simulink model "Projet_Final"  (R2024a)
settings: Solver=FixedStepAuto  StartTime=0.0  StopTime=6  FixedStep=Ts  RelTol=1e-3
values from neighbouring files (symbols this model uses):
  A1 = 0.548    [Parameters.m]
  A2 = 116    [Parameters.m]
  A3 = 0.4    [Parameters.m]
  A4 = 5    [Parameters.m]
  A5 = -21    [Parameters.m]
  A6 = 0.0068    [Parameters.m]
  C_Bat = 1e-3    (= 0.001)    [Parameters.m]    (also in Params_Battery_converter.m)
  C_dc = 4.5e-3    (= 0.0045)    [Parameters.m]
  f = 50    [Parameters.m]
  F = 0.0004924    [Parameters.m]
  G = 6.24    [Parameters.m]
  J = J_PMSG    (= 0.2227)    [Parameters.m]
  J_PMSG = 0.2227    [Parameters.m]
  ki_Ibat = 550    [Parameters.m]    (also in Params_Battery_converter.m)
  ki_id_grid = 225    [Parameters.m]
  ki_iq_grid = ki_id_grid    (= 225)    [Parameters.m]
  ki_isd = 13800    [Parameters.m]
  ki_omega = 0.6873    [Parameters.m]
  ki_PLL = 3200    [Parameters.m]
  ki_Q = 0.05    [Parameters.m]
  ki_vdc = C_dc * W_vdc^2    (= 28.8)    [Parameters.m]
  kp_Ibat = 6.28    [Parameters.m]    (also in Params_Battery_converter.m)
  kp_id_grid = 4.5    [Parameters.m]
  kp_iq_grid = kp_id_grid    (= 4.5)    [Parameters.m]
  kp_isd = 2.75    [Parameters.m]
  kp_omega = 3.108    [Parameters.m]
  kp_PLL = 180    [Parameters.m]
  kp_Q = 0.0005    [Parameters.m]
  kp_vdc = 2 * C_dc * W_vdc    (= 0.72)    [Parameters.m]
  Kt = 1.5 * p * Phi_r    (= 0.7164)    [Parameters.m]
  L_Bat = 2e-3    (= 0.002)    [Parameters.m]    (also in Params_Battery_converter.m)
  Lf = 8e-3    (= 0.008)    [Parameters.m]
  Ls = 0.000395    [Parameters.m]
  p = 4    [Parameters.m]
  Phi_r = 0.1194    [Parameters.m]
  R = 3.96    [Parameters.m]
  Rf = 0.01    [Parameters.m]
  rho = 1.225    [Parameters.m]
  Rs = 0.0485    [Parameters.m]
  S = pi*R^2    (= 49.2651993565)    [Parameters.m]
  Ts = 1e-6    (= 1e-06)    [Parameters.m]
  Vdc_ref = 700    [Parameters.m]    (also in Params_Battery_converter.m)
undefined symbols (not defined in the file or in its folder): Ion, Lithium
libraries: spsSeriesRLCBranchLib x19, slpidlib x11, spsMeanLib x6, spsThreePhaseVIMeasurementLib x6, spsThreePhaseBreakerLib x6, spsIdealSwitchLib x4, spsThreePhaseParallelRLCLoadLib x4, spsCurrentMeasurementLib x3, eeTransforms x3, spsPWMGenerator2LevelLib x3, spsVoltageMeasurementLib x3, spsUniversalBridgeLib x2
(part 1 of 3)
settings Model: SimulationMode=accelerator  Creator=K Edd Edd  LastModifiedBy=K Edd Edd
settings DataIOCC: SignalLogging=off  DSMLogging=off  ReturnWorkspaceOutputs=off

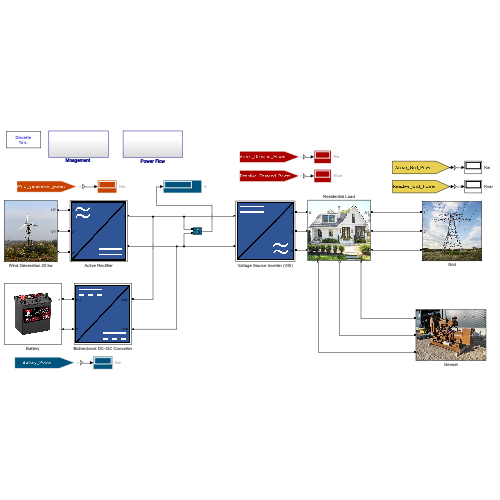
[thumbnail: Simulink's stored preview of the top-level diagram]
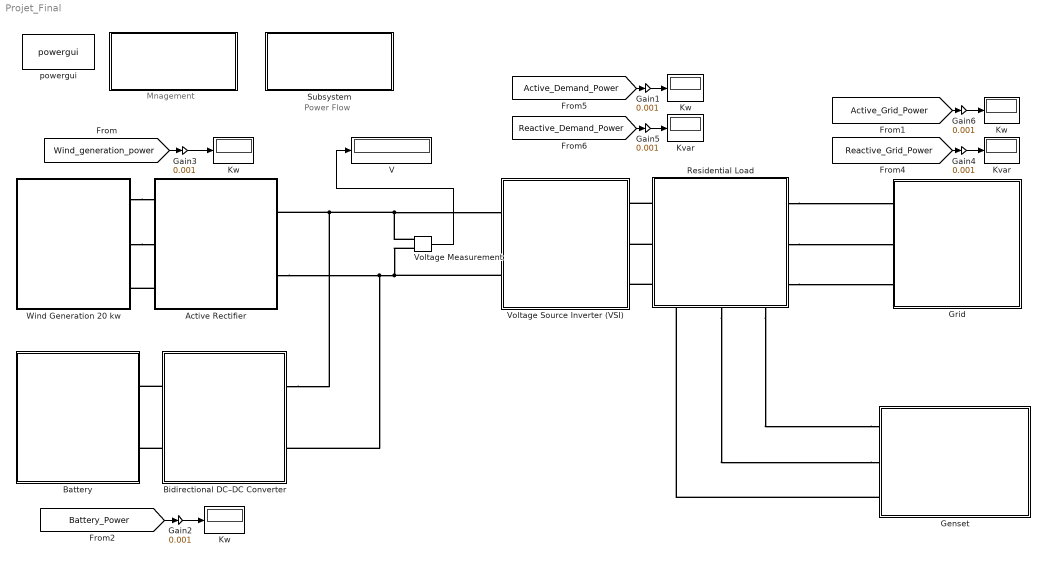
== system Projet_Final ==
  note: Mnagement
  note: Power Flow
  "    " : Subsystem
  Active Rectifier : Subsystem
      mask Display: image('AC-DC converter.png');
  Battery : Subsystem
      mask Display: image('Batterie.jpg', [0,0,0,0,90,90]);
  Bidirectional DC–DC Converter : Subsystem
      mask Display: image('DC-DC converter.png');
  Gain{1..6} (6 alike) : Gain  Gain=0.001
  Genset : Subsystem
      mask Display: image('Cummins-140-kVA-Leroy-Somer-generatorset-Netherlands_8218_1779787131390.jpg');
  Grid : Subsystem
      mask Display: image('df15ac89cc852b7c79e11306f20382d1.jpg');
  Kvar : Display
      settings: Format=bank
  "Kvar  " : Display
      settings: Format=bank
  Kw : Display
      settings: Format=bank
  "Kw  " : Display
      settings: Format=bank
  "Kw   " : Display
      settings: Format=bank
  "Kw    " : Display
      settings: Format=bank
  Residential Load : Subsystem
      settings: PortSchema="{\"entries\":[{\"content\":{\"sides\":[{\"content\":{\"connectorIds\":[\"LConn1\",\"LConn2\",\"LConn3\"]},\"type\":\"ConnectorPlacement.EquallySpacedRectSide\",\"uuid\":\"15385e33-3697-4ec0-8f2e-b1014489e4b6\"},{\"content\":{\"connectorIds\":[\"RConn1\",\"RConn2\",\"RConn3\"],\"side\":\"RIGHT\"},\"type\":\"ConnectorPlacement.EquallySpacedRectSide\",\"uuid\":\"d6a0931e-fc44-44c1-903e-3bbebba5ba41\"},{\"content\":{\"side\":\"TOP\"},\"type\":\"ConnectorPlacement.EquallySpacedRectSide\",\"uuid\":\"1d080c2c-00e5-4060-a5ce-b97d059839f9\"},{\"content\":{\"connectorIds\":[\"RConn4\",\"RConn5\",\"RConn6\"],\"side\":\"BOTTOM\"},\"type\":\"ConnectorPlacement.EquallySpacedRectSide\",\"uuid\":\"92a56d4a-46c7-4b37-87a4-59d3c02e3066\"}]},\"type\":\"ConnectorPlacement.EquallySpacedConnector\",\"uuid\":\"422ce4c9-7dd0-497d-8c7c-a95a054bb062\"}],\"packageUris\":[\"http://schema.mathworks.com/mf0/Connector/R2020b\"],\"version\":\"1.0\"}"
      mask Display: image('home.jpeg');
  Subsystem : Subsystem
  V : Display
      settings: Format=bank
  Voltage Measurement : spsVoltageMeasurementLib/Voltage Measurement  PhasorSimulation=off  OutputType=Complex  PSBequivalent=0
  Voltage Source Inverter (VSI) : Subsystem
      mask Display: image('DC-AC converter.png');
  Wind Generation 20 kw : Subsystem
      mask Display: image('Wind_Turbine.jpg');
  powergui : spspowerguiLib/powergui  Priority=1  SimulationMode=Discrete  SampleTime=Ts  frequency=60  Iterations=50  frequencyindice=0  Pbase=100e6  ErrMax=1e-4  UnitsV=kV  UnitsW=MW  buscounter=0  FunctionMessages=off  echomessages=off  EnableUseOfTLC=off  CurrentSourceSwitches=off  DisableSnubberDevices=off  DisableRonSwitches=off  DisableVfSwitches=off  DisplayEquations=off  AutomaticDiscreteSolvers=off  SolverType=Tustin/Backward Euler (TBE)  Interpol=off  ExternalGateDelay=off  methode=off  Ts=100  x0status=blocks  SPID=on  SwTol=0  HookPort=off  NonlinearTolerance=1e-4  nMaxIteration=100  ContinueOnMaxIteration=off  RestoreLinks=warning  ResistiveCurrentMeasurement=off  Frange=[0:2:500]  Ylog=off  Xlog=on  ShowGrid=off  save=off  variable=ZData  structure=0  ZoomFFT=off  StartTime=0.0  cycles=1  DisplayStyle=1  fundamental=60  FreqAxis=off  MaxFrequency=1000  frequencyindicesteady=1  RmsSteady=1  display=off
  wires:
  Voltage Measurement/1 -> V/1
  Gain3/1 -> Kw/1
  [Wind_generation_power] -> Gain3/1
  Gain2/1 -> "Kw  "/1
  [Battery_Power] -> Gain2/1
  [Reactive_Grid_Power] -> Gain4/1
  [Active_Grid_Power] -> Gain6/1
  Gain5/1 -> Kvar/1
  Gain1/1 -> "Kw   "/1
  [Active_Demand_Power] -> Gain1/1
  [Reactive_Demand_Power] -> Gain5/1
  Gain6/1 -> "Kw    "/1
  Gain4/1 -> "Kvar  "/1
  connections:
  Wind Generation 20 kw/RConn1 -- Active Rectifier/LConn1
  Active Rectifier/LConn3 -- Wind Generation 20 kw/RConn3
  Residential Load/RConn3 -- Grid/LConn3
  Voltage Measurement/LConn1 -- Voltage Source Inverter (VSI)/LConn1 -- Bidirectional DC–DC Converter/LConn1 -- Active Rectifier/RConn1
  Voltage Source Inverter (VSI)/LConn2 -- Active Rectifier/RConn2 -- Bidirectional DC–DC Converter/LConn2 -- Voltage Measurement/LConn2
  Wind Generation 20 kw/RConn2 -- Active Rectifier/LConn2
  Bidirectional DC–DC Converter/RConn1 -- Battery/RConn1
  Bidirectional DC–DC Converter/RConn2 -- Battery/RConn2
  Residential Load/RConn1 -- Grid/LConn1
  Residential Load/RConn2 -- Grid/LConn2
  Residential Load/LConn2 -- Voltage Source Inverter (VSI)/RConn2
  Residential Load/LConn1 -- Voltage Source Inverter (VSI)/RConn1
  Residential Load/LConn3 -- Voltage Source Inverter (VSI)/RConn3
  Genset/RConn3 -- Residential Load/RConn4
  Residential Load/RConn5 -- Genset/RConn2
  Residential Load/RConn6 -- Genset/RConn1

== system Projet_Final/     ==
  Constant{,1..3,5} (5 alike) : Constant
  Constant6 : Constant  Value=0
  tag scope: Cmd_Breaker_Disel=global, Cmd_Breaker_Grid=global, Enable_PWM_GSC=global, Enable_PWM_MSC=global, Enable_Sync=global, Mode_Injection_GSC=global
  wires:
  Constant/1 -> [Cmd_Breaker_Grid]
  Constant1/1 -> [Enable_PWM_GSC]
  Constant2/1 -> [Mode_Injection_GSC]
  Constant3/1 -> [Enable_PWM_MSC]
  Constant6/1 -> [Cmd_Breaker_Disel]
  Constant5/1 -> [Enable_Sync]

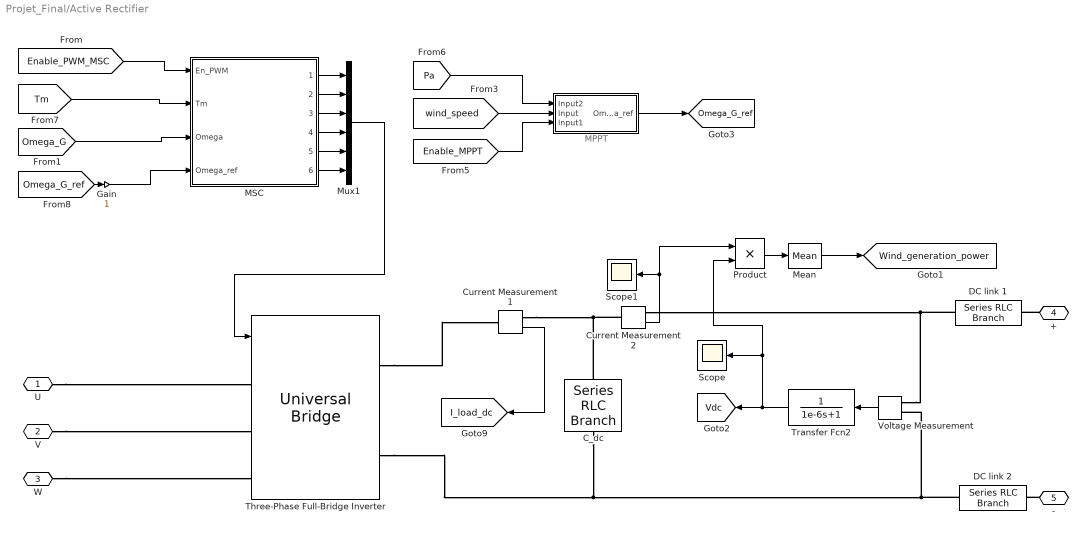
== system Projet_Final/Active Rectifier ==
  note: MPPT
  "      " : Subsystem
  C_dc : spsSeriesRLCBranchLib/Series RLC Branch  LConnTagsString=__new0  RConnTagsString=__new0  BranchType=C  Resistance=0  Inductance=1e-3  SetiL0=off  InitialCurrent=0  Capacitance=C_dc  Setx0=on  InitialVoltage=Vdc_ref  Measurements=None
  Current Measurement1 : spsCurrentMeasurementLib/Current Measurement  PhasorSimulation=off  OutputType=Complex  PSBequivalent=0
  Current Measurement2 : spsCurrentMeasurementLib/Current Measurement  PhasorSimulation=off  OutputType=Complex  PSBequivalent=0
  DC link 1 : spsSeriesRLCBranchLib/Series RLC Branch  LConnTagsString=__new0  RConnTagsString=__new0  BranchType=RL  Resistance=0.01  Inductance=1e-12  SetiL0=off  InitialCurrent=0  Capacitance=C_dc  Setx0=on  InitialVoltage=Vdc_ref  Measurements=None
  DC link 2 : spsSeriesRLCBranchLib/Series RLC Branch  LConnTagsString=__new0  RConnTagsString=__new0  BranchType=RL  Resistance=0.01  Inductance=1e-12  SetiL0=off  InitialCurrent=0  Capacitance=C_dc  Setx0=on  InitialVoltage=Vdc_ref  Measurements=None
  Gain : Gain
  MSC : Subsystem
      settings: PortSchema="{\"entries\":[{\"content\":{\"sides\":[{\"content\":{},\"type\":\"ConnectorPlacement.EquallySpacedRectSide\",\"uuid\":\"68bdff09-e8ec-4d6d-b05e-55201ee357f5\"},{\"content\":{\"side\":\"RIGHT\"},\"type\":\"ConnectorPlacement.EquallySpacedRectSide\",\"uuid\":\"a14a2bca-9db8-408e-b5bf-8e3869a2fb13\"},{\"content\":{\"connectorIds\":[\"Out1\",\"Out2\",\"Out3\",\"Out4\",\"Out5\",\"Out6\"],\"side\":\"TOP\"},\"type\":\"ConnectorPlacement.EquallySpacedRectSide\",\"uuid\":\"600d12f1-b4e8-4864-955c-a539efb19c99\"},{\"content\":{\"connectorIds\":[\"In1\",\"In2\",\"In3\",\"In4\"],\"side\":\"BOTTOM\"},\"type\":\"ConnectorPlacement.EquallySpacedRectSide\",\"uuid\":\"fe719057-0520-4d41-a82f-92eb49034055\"}]},\"type\":\"ConnectorPlacement.EquallySpacedConnector\",\"uuid\":\"05b2b3d9-6bdc-4d72-9457-a6c68afa543f\"}],\"packageUris\":[\"http://schema.mathworks.com/mf0/Connector/R2020b\"],\"version\":\"1.0\"}"
      mask Display: image('Cotroller.jpg', [0,0,0,0,70,70]);
  Mean : spsMeanLib/Mean  Freq=50  Vinit=0  Ts=0
  Mux1 : Mux  Inputs=6
  Product : Product
  Scope : Scope
  Scope1 : Scope
  Three-Phase Full-Bridge Inverter : spsUniversalBridgeLib/Universal Bridge  Arms=3  SnubberResistance=1e7  SnubberCapacitance=inf  Device=IGBT / Diodes  Ron=1e-2  Lon=0  ForwardVoltages="[  0  0  ]"  ForwardVoltage=0  GTOparameters=[ 10e-6 , 20e-6 ]  IGBTparameters=[ 0 , 0 ]  Measurements=None  Measurements_2=None  converterType=Rectifier
  Transfer Fcn2 : TransferFcn  Denominator=[1e-6 1]
  Voltage Measurement : spsVoltageMeasurementLib/Voltage Measurement  PhasorSimulation=off  OutputType=Complex  PSBequivalent=0
  U : PMIOPort  Side=Left
  V : PMIOPort  Port=2  Side=Left
  W : PMIOPort  Port=3  Side=Left
  + : PMIOPort  Port=4  Side=Right
  - : PMIOPort  Port=5  Side=Right
  tag scope: I_load_dc=global, Omega_G_ref=global, Vdc=global, Wind_generation_power=global
  wires:
  Mux1/1 -> Three-Phase Full-Bridge Inverter/1
  [Omega_G_ref] -> Gain/1
  [Tm] -> MSC/2(Tm)
  MSC/3("   ") -> Mux1/3
  MSC/1(" ") -> Mux1/1
  MSC/4("    ") -> Mux1/4
  MSC/6("       ") -> Mux1/6
  MSC/5("     ") -> Mux1/5
  [Omega_G] -> MSC/3(Omega)
  MSC/2("  ") -> Mux1/2
  Voltage Measurement/1 -> Transfer Fcn2/1
  Current Measurement2/1 -> Scope1/1, Product/1
  Current Measurement1/1 -> [I_load_dc]
  Product/1 -> Mean/1
  Mean/1 -> [Wind_generation_power]
  [Enable_PWM_MSC] -> MSC/1(En_PWM)
  "      "/1(Omega_ref) -> [Omega_G_ref]
  [wind_speed] -> "      "/2(Input)
  [Enable_MPPT] -> "      "/3(Input1)
  [Pa] -> "      "/1(Input2)
  Transfer Fcn2/1 -> [Vdc], Scope/1, Product/2
  Gain/1 -> MSC/4(Omega_ref)
  connections:
  V/RConn1 -- Three-Phase Full-Bridge Inverter/LConn2
  U/RConn1 -- Three-Phase Full-Bridge Inverter/LConn1
  W/RConn1 -- Three-Phase Full-Bridge Inverter/LConn3
  C_dc/RConn1 -- Three-Phase Full-Bridge Inverter/RConn2 -- DC link 2/LConn1 -- Voltage Measurement/LConn2
  Current Measurement2/LConn1 -- C_dc/LConn1 -- Current Measurement1/RConn1
  Three-Phase Full-Bridge Inverter/RConn1 -- Current Measurement1/LConn1
  Voltage Measurement/LConn1 -- DC link 1/LConn1 -- Current Measurement2/RConn1
  +/RConn1 -- DC link 1/RConn1
  -/RConn1 -- DC link 2/RConn1

== system Projet_Final/Battery ==
  Battery Status : Scope  NumInputPorts=4
  Battery1 : spsBatteryLib/Battery  BatType=Lithium-Ion  ShowTempParam=off  ThermalPreset=no  ShowAgeParam=off  NomV=450  NomQ=40  SOC=70  Batt_Tr=0.2  PresetModel=on  MaxQ=40  MinV=337.5  FullV=523.7942  Dis_rate=17.3913  R=0.1125  Normal_OP=36.1739  expZone="[486.1736      1.965217]"  current=[1.5 3]  Units=Ampere-hour  Tci=20  NomT=25  T2=0  MaxQ2=2.208  FullV2=3.45  Normal_OP2=2.8  expZone2="[3.22        0.23]"  Rca=0.6  ti=1000  Dp=0  Neq0=0  Tsim=1e6  Ta1=25  Qeol=5.4*0.9  Reol=0.013333*1.2  Char_age=[2.3478, 3]  Dis_age=[2.3478, 10]  N1=1500  N2=10500  N3=1000  N4=1400  Ta2=45  N5=950
      settings: LibrarySourceBlock=electricdrivelib/Extra Sources/Battery
  Bus Selector : BusSelector  OutputSignals=SOC (%),Current (A),Voltage (V)
  Display4 : Display
      settings: Format=bank
  Product1 : Product  RndMeth=Zero
  + : PMIOPort  Side=Right
  - : PMIOPort  Port=2  Side=Right
  tag scope: SOC=global
  wires:
  Product1/1 -> Battery Status/4  "Power_Battery[W]"
  Bus Selector/2 -> Product1/1, Battery Status/2  "<Current (A)>"
  Battery1/1 -> Bus Selector/1
  Bus Selector/3 -> Product1/2, Battery Status/3  "<Voltage (V)>"
  Bus Selector/1 -> Display4/1, [SOC], Battery Status/1  "<SOC (%)>"
  connections:
  Battery1/LConn2 -- -/RConn1
  Battery1/LConn1 -- +/RConn1

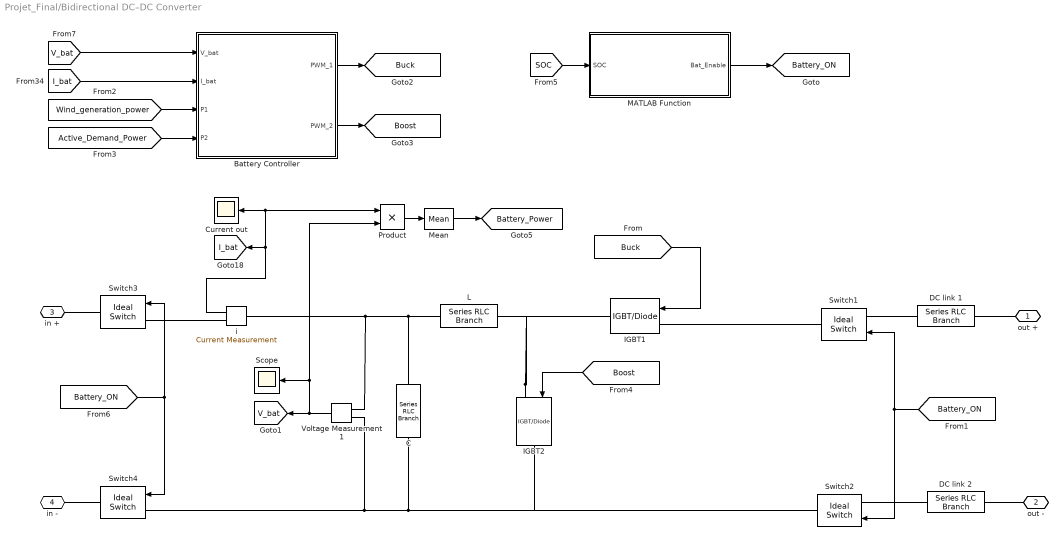
== system Projet_Final/Bidirectional DC–DC Converter ==
  Battery Controller : Subsystem
      mask Display: image('uC.png', [0,0,0,0,70,70]);
  C : spsSeriesRLCBranchLib/Series RLC Branch  LConnTagsString=__new0  RConnTagsString=__new0  BranchType=RC  Resistance=0.00001  Inductance=1e-3  SetiL0=off  InitialCurrent=0  Capacitance=C_Bat  Setx0=off  InitialVoltage=0  Measurements=None
  Current out : Scope
  DC link 1 : spsSeriesRLCBranchLib/Series RLC Branch  LConnTagsString=__new0  RConnTagsString=__new0  BranchType=RL  Resistance=0.01  Inductance=1e-12  SetiL0=off  InitialCurrent=0  Capacitance=C_dc  Setx0=on  InitialVoltage=Vdc_ref  Measurements=None
  DC link 2 : spsSeriesRLCBranchLib/Series RLC Branch  LConnTagsString=__new0  RConnTagsString=__new0  BranchType=RL  Resistance=0.01  Inductance=1e-12  SetiL0=off  InitialCurrent=0  Capacitance=C_dc  Setx0=on  InitialVoltage=Vdc_ref  Measurements=None
  IGBT1 : spsIGBTDiodeLib/IGBT//Diode  Ron=1e-3  Rs=1e5  Cs=inf  Measurements=off
  IGBT2 : spsIGBTDiodeLib/IGBT//Diode  Ron=1e-3  Rs=1e5  Cs=inf  Measurements=off
  L : spsSeriesRLCBranchLib/Series RLC Branch  LConnTagsString=__new0  RConnTagsString=__new0  BranchType=RL  Resistance=0.00001  Inductance=L_Bat  SetiL0=off  InitialCurrent=0  Capacitance=1000e-6  Setx0=off  InitialVoltage=0  Measurements=None
  MATLAB Function : MATLAB Function  TreatAsAtomicUnit=on
  Mean : spsMeanLib/Mean  Freq=50  Vinit=0  Ts=0
  Product : Product
  Scope : Scope
  Switch{1..4} (4 alike) : spsIdealSwitchLib/Ideal Switch  Ron=0.001  Lon=0  IC=0  Rs=1e6  Cs=inf  Measurements=off
  Voltage Measurement1 : spsVoltageMeasurementLib/Voltage Measurement  PhasorSimulation=off  OutputType=Complex  PSBequivalent=0
  i : spsCurrentMeasurementLib/Current Measurement  PhasorSimulation=off  OutputType=Complex  PSBequivalent=0
  out + : PMIOPort  Side=Left
  out - : PMIOPort  Port=2  Side=Left
  in + : PMIOPort  Port=3  Side=Right
  in - : PMIOPort  Port=4  Side=Right
  tag scope: Battery_ON=global, Battery_Power=global, Boost=global, Buck=global, I_bat=global, V_bat=global
  wires:
  [Buck] -> IGBT1/1
  MATLAB Function/1(Bat_Enable) -> [Battery_ON]
  [Wind_generation_power] -> Battery Controller/3(P1)
  Battery Controller/1(PWM_1) -> [Buck]
  [Battery_ON] -> Switch4/1, Switch3/1
  Mean/1 -> [Battery_Power]
  Battery Controller/2(PWM_2) -> [Boost]
  [Active_Demand_Power] -> Battery Controller/4(P2)
  Product/1 -> Mean/1
  [Boost] -> IGBT2/1
  [I_bat] -> Battery Controller/2(I_bat)
  Voltage Measurement1/1 -> Product/2, Scope/1, [V_bat]
  [Battery_ON] -> Switch1/1, Switch2/1
  [V_bat] -> Battery Controller/1(V_bat)
  [SOC] -> MATLAB Function/1(SOC)
  i/1 -> Product/1, Current out/1, [I_bat]
  connections:
  Switch3/RConn1 -- in +/RConn1
  Switch4/RConn1 -- in -/RConn1
  i/RConn1 -- Switch3/LConn1
  IGBT2/LConn1 -- L/RConn1 -- IGBT1/RConn1
  IGBT1/LConn1 -- Switch1/RConn1
  Voltage Measurement1/LConn1 -- C/LConn1 -- L/LConn1 -- i/LConn1
  DC link 1/RConn1 -- out +/RConn1
  DC link 2/LConn1 -- Switch2/LConn1
  Voltage Measurement1/LConn2 -- Switch2/RConn1 -- IGBT2/RConn1 -- C/RConn1 -- Switch4/LConn1
  Switch1/LConn1 -- DC link 1/LConn1
  out -/RConn1 -- DC link 2/RConn1

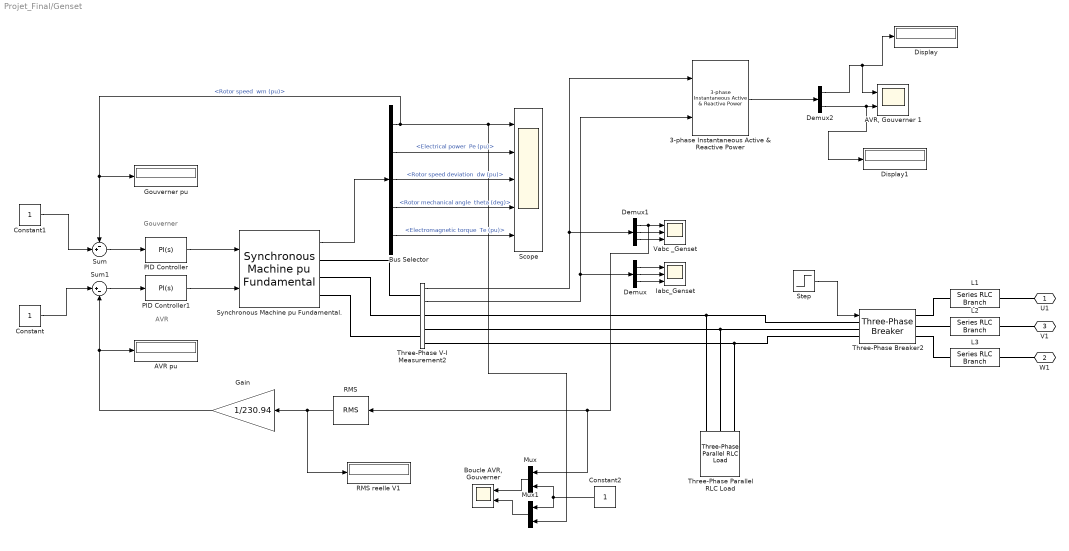
== system Projet_Final/Genset ==
  note: AVR
  note: Gouverner
  3-phase Instantaneous Active & Reactive Power : powerlib_extras/Measurements/3-phase  Instantaneous  Active & Reactive Power
  AVR pu : Display
  "AVR, Gouverner 1" : Scope  NumInputPorts=2
  "Boucle AVR, Gouverner " : Scope  NumInputPorts=2
  Bus Selector : BusSelector  OutputSignals="Mechanical.Rotor speed  wm (pu),Mechanical.Electrical power  Pe (pu),Mechanical.Rotor speed deviation  dw (pu),Mechanical.Rotor mechanical angle  theta (deg),Mechanical.Electromagnetic torque  Te (pu)"
  Constant : Constant
  Constant1 : Constant
  Constant2 : Constant
  Demux : Demux  Outputs=3
  Demux1 : Demux  Outputs=3
  Demux2 : Demux  Outputs=2
  Display : Display
      settings: Format=bank
  Display1 : Display
      settings: Format=bank
  Gain : Gain  Gain=1/230.94
  Gouverner pu : Display
  Iabc_Genset : Scope  NumInputPorts=3
  L1 : spsSeriesRLCBranchLib/Series RLC Branch  LConnTagsString=__new0  RConnTagsString=__new0  BranchType=RL  Resistance=0.01  Inductance=1e-12  SetiL0=off  InitialCurrent=0  Capacitance=C_dc  Setx0=on  InitialVoltage=Vdc_ref  Measurements=None
  L2 : spsSeriesRLCBranchLib/Series RLC Branch  LConnTagsString=__new0  RConnTagsString=__new0  BranchType=RL  Resistance=0.01  Inductance=1e-12  SetiL0=off  InitialCurrent=0  Capacitance=C_dc  Setx0=on  InitialVoltage=Vdc_ref  Measurements=None
  L3 : spsSeriesRLCBranchLib/Series RLC Branch  LConnTagsString=__new0  RConnTagsString=__new0  BranchType=RL  Resistance=0.01  Inductance=1e-12  SetiL0=off  InitialCurrent=0  Capacitance=C_dc  Setx0=on  InitialVoltage=Vdc_ref  Measurements=None
  Mux : Mux  Inputs=2
  Mux1 : Mux  Inputs=2
  PID Controller : slpidlib/PID Controller  Controller=PI  Form=Parallel  TimeDomain=Continuous-time  UseExternalTs=off  SampleTime=-1  IntegratorMethod=Forward Euler  FilterMethod=Forward Euler  ControllerParametersSource=internal  P=50  I=40  UseKiTs=off  D=0  UseExternalDerivativeSource=off  N=100  UseFilter=on  TunerSelectOption=Transfer Function Based (PID Tuner App)  InitialConditionSource=internal  InitialConditionForIntegrator=0.0205767  InitialConditionForFilter=0  DifferentiatorICPrevScaledInput=0  ExternalReset=none  TrackingMode=off  Kt=1  LimitOutput=on  SatLimitsSource=internal  UpperSaturationLimit=1.1  LowerSaturationLimit=0  LinearizeAsGain=on  AntiWindupMode=none  Kb=1  LimitIntegrator=off  UpperIntegratorSaturationLimit=inf  LowerIntegratorSaturationLimit=-inf  POutMin=[]  POutMax=[]  IOutMin=[]  IOutMax=[]  DOutMin=[]  DOutMax=[]  NOutMin=[]  NOutMax=[]  SumOutMin=[]  SumOutMax=[]  SaturationOutMin=[]  SaturationOutMax=[]  PParamMin=[]  PParamMax=[]  IParamMin=[]  IParamMax=[]  DParamMin=[]  DParamMax=[]  NParamMin=[]  NParamMax=[]  KbParamMin=[]  KbParamMax=[]  KtParamMin=[]  KtParamMax=[]  KbOutMin=[]  KbOutMax=[]  KtOutMin=[]  KtOutMax=[]  IntegratorOutMin=[]  IntegratorOutMax=[]  FilterOutMin=[]  FilterOutMax=[]  SumI1OutMin=[]  SumI1OutMax=[]  SumI2OutMin=[]  SumI2OutMax=[]  SumI3OutMin=[]  SumI3OutMax=[]  SumI4OutMin=[]  SumI4OutMax=[]  SumDOutMin=[]  SumDOutMax=[]  DifferentiatorOutMin=[]  DifferentiatorOutMax=[]  FilterDiffOutCoefMin=[]  FilterDiffOutCoefMax=[]  ReciprocalOutMin=[]  ReciprocalOutMax=[]  SumDenOutMin=[]  SumDenOutMax=[]  SumNumOutMin=[]  SumNumOutMax=[]  DivideOutMin=[]  DivideOutMax=[]  UdiffTsProdOutMin=[]  UdiffTsProdOutMax=[]  NTsProdOutMin=[]  NTsProdOutMax=[]  UintegralTsProdOutMin=[]  UintegralTsProdOutMax=[]  UngainTsProdOutMin=[]  UngainTsProdOutMax=[]  ClampingZeroOutDataTypeStr=Inherit: Inherit via back propagation  ClampingZeroOutMin=[]  ClampingZeroOutMax=[]  FilterDenConstantOutDataTypeStr=Inherit: Inherit via back propagation  FilterDenConstantOutMin=[]  FilterDenConstantOutMax=[]  PCopyOutDataTypeStr=Inherit: Inherit via back propagation  PCopyOutMin=[]  PCopyOutMax=[]  NCopyOutDataTypeStr=Inherit: Inherit via back propagation  NCopyOutMin=[]  NCopyOutMax=[]  IntegratorContinuousStateAttributes=''  IntegratorStateMustResolveToSignalObject=off  IntegratorRTWStateStorageClass=Auto  FilterContinuousStateAttributes=''  FilterStateMustResolveToSignalObject=off  FilterRTWStateStorageClass=Auto  ParallelPVariant=InternalParameters  IdealPVariant=Disabled  IVariant=InternalParameters  DVariant=Disabled  IntegratorVariant=Continuous  SatVariant=Enabled  AWVariant=Passthrough  PCopyVariant=Disabled  TRVariant=Disabled  FdbkBlocksVariant=Forward  IdealPFdbkVariant=Disabled  SatFdbkVariant=Disabled  DerivativeFilterVariant=Disabled  NVariant=Disabled  NCopyVariant=Disabled_SignalSpec  FilterICVariant=Disabled  IntegratorICVariant=InternalICs  ExternalResetVariant=Disabled  TRSumVariant=Passthrough  SumFdbkVariant=Disabled  SumVariant=Sum_PI  TsampFilterVariant=InternalTs  TsampNgainVariant=Passthrough  TsampIntegralVariant=Disabled_SignalSpec  ExternalSaturationOutDataTypeStr=Inherit: Same as second input  DerivativeSourceVariant=Disabled
  PID Controller1 : slpidlib/PID Controller  Controller=PI  Form=Parallel  TimeDomain=Continuous-time  UseExternalTs=off  SampleTime=-1  IntegratorMethod=Forward Euler  FilterMethod=Forward Euler  ControllerParametersSource=internal  P=100  I=20  UseKiTs=off  D=0  UseExternalDerivativeSource=off  N=100  UseFilter=on  TunerSelectOption=Transfer Function Based (PID Tuner App)  InitialConditionSource=internal  InitialConditionForIntegrator=1  InitialConditionForFilter=0  DifferentiatorICPrevScaledInput=0  ExternalReset=none  TrackingMode=off  Kt=1  LimitOutput=on  SatLimitsSource=internal  UpperSaturationLimit=5  LowerSaturationLimit=0  LinearizeAsGain=on  AntiWindupMode=none  Kb=1  LimitIntegrator=off  UpperIntegratorSaturationLimit=inf  LowerIntegratorSaturationLimit=-inf  POutMin=[]  POutMax=[]  IOutMin=[]  IOutMax=[]  DOutMin=[]  DOutMax=[]  NOutMin=[]  NOutMax=[]  SumOutMin=[]  SumOutMax=[]  SaturationOutMin=[]  SaturationOutMax=[]  PParamMin=[]  PParamMax=[]  IParamMin=[]  IParamMax=[]  DParamMin=[]  DParamMax=[]  NParamMin=[]  NParamMax=[]  KbParamMin=[]  KbParamMax=[]  KtParamMin=[]  KtParamMax=[]  KbOutMin=[]  KbOutMax=[]  KtOutMin=[]  KtOutMax=[]  IntegratorOutMin=[]  IntegratorOutMax=[]  FilterOutMin=[]  FilterOutMax=[]  SumI1OutMin=[]  SumI1OutMax=[]  SumI2OutMin=[]  SumI2OutMax=[]  SumI3OutMin=[]  SumI3OutMax=[]  SumI4OutMin=[]  SumI4OutMax=[]  SumDOutMin=[]  SumDOutMax=[]  DifferentiatorOutMin=[]  DifferentiatorOutMax=[]  FilterDiffOutCoefMin=[]  FilterDiffOutCoefMax=[]  ReciprocalOutMin=[]  ReciprocalOutMax=[]  SumDenOutMin=[]  SumDenOutMax=[]  SumNumOutMin=[]  SumNumOutMax=[]  DivideOutMin=[]  DivideOutMax=[]  UdiffTsProdOutMin=[]  UdiffTsProdOutMax=[]  NTsProdOutMin=[]  NTsProdOutMax=[]  UintegralTsProdOutMin=[]  UintegralTsProdOutMax=[]  UngainTsProdOutMin=[]  UngainTsProdOutMax=[]  ClampingZeroOutDataTypeStr=Inherit: Inherit via back propagation  ClampingZeroOutMin=[]  ClampingZeroOutMax=[]  FilterDenConstantOutDataTypeStr=Inherit: Inherit via back propagation  FilterDenConstantOutMin=[]  FilterDenConstantOutMax=[]  PCopyOutDataTypeStr=Inherit: Inherit via back propagation  PCopyOutMin=[]  PCopyOutMax=[]  NCopyOutDataTypeStr=Inherit: Inherit via back propagation  NCopyOutMin=[]  NCopyOutMax=[]  IntegratorContinuousStateAttributes=''  IntegratorStateMustResolveToSignalObject=off  IntegratorRTWStateStorageClass=Auto  FilterContinuousStateAttributes=''  FilterStateMustResolveToSignalObject=off  FilterRTWStateStorageClass=Auto  ParallelPVariant=InternalParameters  IdealPVariant=Disabled  IVariant=InternalParameters  DVariant=Disabled  IntegratorVariant=Continuous  SatVariant=Enabled  AWVariant=Passthrough  PCopyVariant=Disabled  TRVariant=Disabled  FdbkBlocksVariant=Forward  IdealPFdbkVariant=Disabled  SatFdbkVariant=Disabled  DerivativeFilterVariant=Disabled  NVariant=Disabled  NCopyVariant=Disabled_SignalSpec  FilterICVariant=Disabled  IntegratorICVariant=InternalICs  ExternalResetVariant=Disabled  TRSumVariant=Passthrough  SumFdbkVariant=Disabled  SumVariant=Sum_PI  TsampFilterVariant=InternalTs  TsampNgainVariant=Passthrough  TsampIntegralVariant=Disabled_SignalSpec  ExternalSaturationOutDataTypeStr=Inherit: Same as second input  DerivativeSourceVariant=Disabled
  RMS : spsRMSLib/RMS  TrueRMS=on  Freq=50  RMSInit=0  Ts=Ts
  RMS reelle V1 : Display
  Scope : Scope  NumInputPorts=5
  Step : Step  Time=0  Before=1  After=0  SampleTime=0
  Sum : Sum  Inputs=-+|
  Sum1 : Sum  Inputs=|+-
  Synchronous Machine pu Fundamental. : spsSynchronousMachinepuFundamentalLib/Synchronous Machine pu Fundamental  PresetModel=No  MechanicalLoad=Mechanical power Pm  ShowDetailedParameters=on  RotorType=Salient-pole  Units=per unit fundamental parameters  MeasurementBus=off  NominalParameters=[6e+04 400 50]  Stator=[0.03788 0.08 2.16 0.94]  Field=[0.02124 0.1719]  Dampers2=[0.0652, 0.5134, 0.0287, 0.2553, 7.765e-3, 0.9167 ]  Dampers1=[0.1463 0.3085 0.05754 0.05281]  Mechanical=[0.1028 0.02056 2]  PolePairs=2  InitialConditions=[0 -89.999 1.66667e-05 1.66667e-05 1.66667e-05 0 -120 120 1]  SetSaturation=off  Saturation=[0.6404,0.7127,0.8441,0.9214,0.9956,1.082,1.19,1.316,1.457;0.7,0.7698,0.8872,0.9466,0.9969,1.046,1.1,1.151,1.201]  LoadFlowParameters=[2 1 0 0 0]  TsPowergui=0  TsBlock=-1  IterativeModel=Trapezoidal non iterative  IterativeDiscreteModel=Trapezoidal non iterative  BusType=PV  Pref=20000  Qref=0  Qmin=-inf  Qmax=inf  PLF=0  QLF=0
      settings: LibrarySourceBlock=|
      | sps_lib/Electrical Machines/Synchronous Machine
      | pu Fundamental
  Three-Phase Parallel RLC Load : spsThreePhaseParallelRLCLoadLib/Three-Phase Parallel RLC Load  LConnTagsString=A|B|C  Configuration=Y (grounded)  NominalVoltage=400  Vabc=[1e3 1e3 1e3]  Vabcp=[1e3 1e3 1e3]  NominalFrequency=50  UnbalancedPower=off  ActivePower=1234.6  InductivePower=0  CapacitivePower=0  Pabc=[10e3 9e3 11e3]  QLabc=[100 90 110]  QCabc=[100 90 110]  Pabcp=[10e3 9e3 11e3]  QLabcp=[100 90 110]  QCabcp=[100 90 110]  Measurements=None  LoadType=constant PQ
  Three-Phase V-I Measurement2 : spsThreePhaseVIMeasurementLib/Three-Phase V-I Measurement  VoltageMeasurement=phase-to-ground  SetLabelV=off  LabelV=Vabc_Inverter  Vpu=off  VpuLL=off  CurrentMeasurement=yes  SetLabelI=off  LabelI=Iabc_Inverter  Ipu=off  Pbase=100e6  Vbase=500e3  OutputType=Complex  PhasorSimulation=off  PSBequivalent=0
  Three-Phase Breaker2 : spsThreePhaseBreakerLib/Three-Phase Breaker  InitialState=open  SwitchA=on  SwitchB=on  SwitchC=on  SwitchTimes="[1/60  5/60]"  External=on  BreakerResistance=0.01  SnubberResistance=1e6  SnubberCapacitance=inf  Measurements=None
  Vabc _Genset : Scope  NumInputPorts=3
  U1 : PMIOPort  Side=Right
  W1 : PMIOPort  Port=2  Side=Right
  V1 : PMIOPort  Port=3  Side=Right
  wires:
  Step/1 -> Three-Phase Breaker2/1
  3-phase Instantaneous Active & Reactive Power/1 -> Demux2/1
  Bus Selector/5 -> Scope/5  "<Electromagnetic torque  Te (pu)>"
  Gain/1 -> Sum1/2, AVR pu/1
  Demux/2 -> Iabc_Genset/2
  Bus Selector/4 -> Scope/4  "<Rotor mechanical angle  theta (deg)>"
  Constant1/1 -> Sum/2
  Demux/1 -> Iabc_Genset/1
  Constant/1 -> Sum1/1
  Bus Selector/1 -> Gouverner pu/1, Sum/1, Mux1/2, Scope/1  "<Rotor speed  wm (pu)>"
  Demux1/2 -> Vabc _Genset/2
  Synchronous Machine pu Fundamental./1 -> Bus Selector/1
  Mux1/1 -> "Boucle AVR, Gouverner "/2
  Sum/1 -> PID Controller/1
  Demux1/1 -> Mux/1, RMS/1, Vabc _Genset/1
  Bus Selector/2 -> Scope/2  "<Electrical power  Pe (pu)>"
  Bus Selector/3 -> Scope/3  "<Rotor speed deviation  dw (pu)>"
  Demux1/3 -> Vabc _Genset/3
  Mux/1 -> "Boucle AVR, Gouverner "/1
  Constant2/1 -> Mux1/1, Mux/2
  RMS/1 -> RMS reelle V1/1, Gain/1
  Demux/3 -> Iabc_Genset/3
  Three-Phase V-I Measurement2/1 -> 3-phase Instantaneous Active & Reactive Power/1, Demux1/1
  PID Controller1/1 -> Synchronous Machine pu Fundamental./2
  Three-Phase V-I Measurement2/2 -> 3-phase Instantaneous Active & Reactive Power/2, Demux/1
  Demux2/2 -> Display1/1, "AVR, Gouverner 1"/2
  Sum1/1 -> PID Controller1/1
  Demux2/1 -> Display/1, "AVR, Gouverner 1"/1
  PID Controller/1 -> Synchronous Machine pu Fundamental./1
  connections:
  Three-Phase V-I Measurement2/LConn1 -- Synchronous Machine pu Fundamental./RConn1
  Three-Phase V-I Measurement2/LConn3 -- Synchronous Machine pu Fundamental./RConn3
  Three-Phase V-I Measurement2/LConn2 -- Synchronous Machine pu Fundamental./RConn2
  Three-Phase V-I Measurement2/RConn1 -- Three-Phase Breaker2/LConn1 -- Three-Phase Parallel RLC Load/LConn1
  Three-Phase V-I Measurement2/RConn2 -- Three-Phase Parallel RLC Load/LConn2 -- Three-Phase Breaker2/LConn2
  Three-Phase V-I Measurement2/RConn3 -- Three-Phase Breaker2/LConn3 -- Three-Phase Parallel RLC Load/LConn3
  L2/LConn1 -- Three-Phase Breaker2/RConn2
  Three-Phase Breaker2/RConn1 -- L1/LConn1
  L3/LConn1 -- Three-Phase Breaker2/RConn3
  L2/RConn1 -- V1/RConn1
  U1/RConn1 -- L1/RConn1
  W1/RConn1 -- L3/RConn1

== system Projet_Final/Grid ==
  L1 : spsSeriesRLCBranchLib/Series RLC Branch  LConnTagsString=__new0  RConnTagsString=__new0  BranchType=RL  Resistance=0.01  Inductance=1e-12  SetiL0=off  InitialCurrent=0  Capacitance=C_dc  Setx0=on  InitialVoltage=Vdc_ref  Measurements=None
  L2 : spsSeriesRLCBranchLib/Series RLC Branch  LConnTagsString=__new0  RConnTagsString=__new0  BranchType=RL  Resistance=0.01  Inductance=1e-12  SetiL0=off  InitialCurrent=0  Capacitance=C_dc  Setx0=on  InitialVoltage=Vdc_ref  Measurements=None
  L3 : spsSeriesRLCBranchLib/Series RLC Branch  LConnTagsString=__new0  RConnTagsString=__new0  BranchType=RL  Resistance=0.01  Inductance=1e-12  SetiL0=off  InitialCurrent=0  Capacitance=C_dc  Setx0=on  InitialVoltage=Vdc_ref  Measurements=None
  Three-Phase Source : spsThreePhaseSourceLib/Three-Phase Source  InternalConnection=Yg  VoltagePhases=off  Voltage=400  PhaseAngle=0  Voltage_phases=[25e3 25e3 25e3]/sqrt(3)  PhaseAngles_phases=[0 -120 +120]  Frequency=50  NonIdealSource=on  SpecifyImpedance=off  Resistance=0.00000001  Inductance=0.00000001  ShortCircuitLevel=100e6  BaseVoltage=400  XRratio=7  BusType=swing  Pref=10e3  Qref=0  Prefabc=[10e3, 10e3, 10e3]  Qrefabc=[0, 0, 0]  Qmin=-inf  Qmax=inf
  1 : PMIOPort  Side=Left
  2 : PMIOPort  Port=2  Side=Left
  3 : PMIOPort  Port=3  Side=Left
  connections:
  L2/RConn1 -- Three-Phase Source/RConn2
  L1/LConn1 -- 1/RConn1
  L3/LConn1 -- 3/RConn1
  2/RConn1 -- L2/LConn1
  Three-Phase Source/RConn1 -- L1/RConn1
  Three-Phase Source/RConn3 -- L3/RConn1

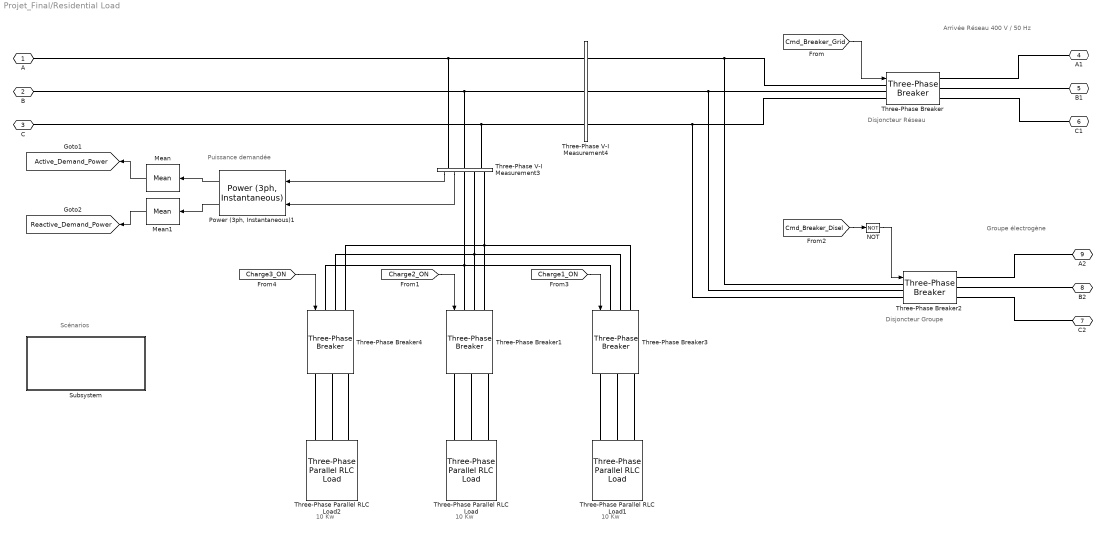
== system Projet_Final/Residential Load ==
  note: Scénarios
  note: Puissance demandée
  note: 10 Kw
  note: 10 Kw
  note: 10 Kw
  note: Arrivée Réseau 400 V / 50 Hz
  note: Groupe électrogène
  note: Disjoncteur Réseau
  note: Disjoncteur Groupe
  Mean : spsMeanLib/Mean  Freq=50  Vinit=0  Ts=0
  Mean1 : spsMeanLib/Mean  Freq=50  Vinit=0  Ts=0
  NOT : Logic  Operator=NOT  IconShape=distinctive  AllPortsSameDT=off  OutDataTypeStr=boolean
  "Power (3ph, Instantaneous)1" : spsPower3phInstantaneousLib/Power (3ph, Instantaneous)
  Subsystem : Subsystem
  Three-Phase Parallel RLC Load : spsThreePhaseParallelRLCLoadLib/Three-Phase Parallel RLC Load  LConnTagsString=A|B|C  Configuration=Y (grounded)  NominalVoltage=400  Vabc=[1e3 1e3 1e3]  Vabcp=[1e3 1e3 1e3]  NominalFrequency=50  UnbalancedPower=off  ActivePower=10000  InductivePower=0  CapacitivePower=0  Pabc=[10e3 9e3 11e3]  QLabc=[100 90 110]  QCabc=[100 90 110]  Pabcp=[10e3 9e3 11e3]  QLabcp=[100 90 110]  QCabcp=[100 90 110]  Measurements=None  LoadType=constant PQ
  Three-Phase Parallel RLC Load1 : spsThreePhaseParallelRLCLoadLib/Three-Phase Parallel RLC Load  LConnTagsString=A|B|C  Configuration=Y (grounded)  NominalVoltage=400  Vabc=[1e3 1e3 1e3]  Vabcp=[1e3 1e3 1e3]  NominalFrequency=50  UnbalancedPower=off  ActivePower=10000  InductivePower=0  CapacitivePower=0  Pabc=[10e3 9e3 11e3]  QLabc=[100 90 110]  QCabc=[100 90 110]  Pabcp=[10e3 9e3 11e3]  QLabcp=[100 90 110]  QCabcp=[100 90 110]  Measurements=None  LoadType=constant PQ
  Three-Phase Parallel RLC Load2 : spsThreePhaseParallelRLCLoadLib/Three-Phase Parallel RLC Load  LConnTagsString=A|B|C  Configuration=Y (grounded)  NominalVoltage=400  Vabc=[1e3 1e3 1e3]  Vabcp=[1e3 1e3 1e3]  NominalFrequency=50  UnbalancedPower=off  ActivePower=10000  InductivePower=0  CapacitivePower=0  Pabc=[10e3 9e3 11e3]  QLabc=[100 90 110]  QCabc=[100 90 110]  Pabcp=[10e3 9e3 11e3]  QLabcp=[100 90 110]  QCabcp=[100 90 110]  Measurements=None  LoadType=constant PQ
  Three-Phase V-I Measurement3 : spsThreePhaseVIMeasurementLib/Three-Phase V-I Measurement  VoltageMeasurement=phase-to-ground  SetLabelV=off  LabelV=Vabc_load  Vpu=off  VpuLL=off  CurrentMeasurement=yes  SetLabelI=off  LabelI=Iabc_load  Ipu=off  Pbase=100e6  Vbase=500e3  OutputType=Complex  PhasorSimulation=off  PSBequivalent=0
  Three-Phase V-I Measurement4 : spsThreePhaseVIMeasurementLib/Three-Phase V-I Measurement  VoltageMeasurement=phase-to-ground  SetLabelV=on  LabelV=Vabc_grid  Vpu=off  VpuLL=off  CurrentMeasurement=yes  SetLabelI=on  LabelI=Iabc_grid  Ipu=off  Pbase=100e6  Vbase=500e3  OutputType=Complex  PhasorSimulation=off  PSBequivalent=0
  Three-Phase Breaker : spsThreePhaseBreakerLib/Three-Phase Breaker  InitialState=open  SwitchA=on  SwitchB=on  SwitchC=on  SwitchTimes="[1/60  5/60]"  External=on  BreakerResistance=0.01  SnubberResistance=1e6  SnubberCapacitance=inf  Measurements=None
  Three-Phase Breaker1 : spsThreePhaseBreakerLib/Three-Phase Breaker  InitialState=open  SwitchA=on  SwitchB=on  SwitchC=on  SwitchTimes="[1/60  5/60]"  External=on  BreakerResistance=0.01  SnubberResistance=1e12  SnubberCapacitance=inf  Measurements=None
  Three-Phase Breaker2 : spsThreePhaseBreakerLib/Three-Phase Breaker  InitialState=open  SwitchA=on  SwitchB=on  SwitchC=on  SwitchTimes="[1/60  5/60]"  External=on  BreakerResistance=0.01  SnubberResistance=1e6  SnubberCapacitance=inf  Measurements=None
  Three-Phase Breaker3 : spsThreePhaseBreakerLib/Three-Phase Breaker  InitialState=open  SwitchA=on  SwitchB=on  SwitchC=on  SwitchTimes="[1/60  5/60]"  External=on  BreakerResistance=0.01  SnubberResistance=1e12  SnubberCapacitance=inf  Measurements=None
  Three-Phase Breaker4 : spsThreePhaseBreakerLib/Three-Phase Breaker  InitialState=open  SwitchA=on  SwitchB=on  SwitchC=on  SwitchTimes="[1/60  5/60]"  External=on  BreakerResistance=0.01  SnubberResistance=1e12  SnubberCapacitance=inf  Measurements=None
  A : PMIOPort  Side=Left
  B : PMIOPort  Port=2  Side=Left
  C : PMIOPort  Port=3  Side=Left
  A1 : PMIOPort  Port=4  Side=Right
  B1 : PMIOPort  Port=5  Side=Right
  C1 : PMIOPort  Port=6  Side=Right
  C2 : PMIOPort  Port=7  Side=Right
  B2 : PMIOPort  Port=8  Side=Right
  A2 : PMIOPort  Port=9  Side=Right
  tag scope: Active_Demand_Power=global, Reactive_Demand_Power=global
  wires:
  [Cmd_Breaker_Grid] -> Three-Phase Breaker/1
  [Cmd_Breaker_Disel] -> NOT/1
  NOT/1 -> Three-Phase Breaker2/1
  Three-Phase V-I Measurement3/1 -> "Power (3ph, Instantaneous)1"/1
  [Charge1_ON] -> Three-Phase Breaker3/1
  [Charge3_ON] -> Three-Phase Breaker4/1
  [Charge2_ON] -> Three-Phase Breaker1/1
  Three-Phase V-I Measurement3/2 -> "Power (3ph, Instantaneous)1"/2
  "Power (3ph, Instantaneous)1"/2 -> Mean1/1
  "Power (3ph, Instantaneous)1"/1 -> Mean/1
  Mean/1 -> [Active_Demand_Power]
  Mean1/1 -> [Reactive_Demand_Power]
  connections:
  Three-Phase Breaker/LConn2 -- Three-Phase V-I Measurement4/RConn2 -- Three-Phase Breaker2/LConn2
  A2/RConn1 -- Three-Phase Breaker2/RConn1
  B2/RConn1 -- Three-Phase Breaker2/RConn2
  C2/RConn1 -- Three-Phase Breaker2/RConn3
  Three-Phase Breaker1/LConn1 -- Three-Phase V-I Measurement3/RConn1 -- Three-Phase Breaker3/LConn1 -- Three-Phase Breaker4/LConn1
  Three-Phase Parallel RLC Load/LConn3 -- Three-Phase Breaker1/RConn3
  Three-Phase Parallel RLC Load/LConn2 -- Three-Phase Breaker1/RConn2
  Three-Phase Parallel RLC Load/LConn1 -- Three-Phase Breaker1/RConn1
  Three-Phase Parallel RLC Load2/LConn1 -- Three-Phase Breaker4/RConn1
  Three-Phase Parallel RLC Load2/LConn2 -- Three-Phase Breaker4/RConn2
  Three-Phase Parallel RLC Load2/LConn3 -- Three-Phase Breaker4/RConn3
  Three-Phase Breaker1/LConn2 -- Three-Phase Breaker4/LConn2 -- Three-Phase V-I Measurement3/RConn2 -- Three-Phase Breaker3/LConn2
  Three-Phase Breaker1/LConn3 -- Three-Phase Breaker3/LConn3 -- Three-Phase V-I Measurement3/RConn3 -- Three-Phase Breaker4/LConn3
  Three-Phase Breaker/RConn3 -- C1/RConn1
  Three-Phase Breaker/RConn2 -- B1/RConn1
  Three-Phase Breaker/RConn1 -- A1/RConn1
  Three-Phase Breaker2/LConn3 -- Three-Phase V-I Measurement4/RConn3 -- Three-Phase Breaker/LConn3
  Three-Phase Breaker/LConn1 -- Three-Phase V-I Measurement4/RConn1 -- Three-Phase Breaker2/LConn1
  Three-Phase Parallel RLC Load1/LConn3 -- Three-Phase Breaker3/RConn3
  Three-Phase Parallel RLC Load1/LConn2 -- Three-Phase Breaker3/RConn2
  Three-Phase Parallel RLC Load1/LConn1 -- Three-Phase Breaker3/RConn1
  Three-Phase V-I Measurement4/LConn3 -- Three-Phase V-I Measurement3/LConn3 -- C/RConn1
  B/RConn1 -- Three-Phase V-I Measurement3/LConn2 -- Three-Phase V-I Measurement4/LConn2
  A/RConn1 -- Three-Phase V-I Measurement3/LConn1 -- Three-Phase V-I Measurement4/LConn1

== system Projet_Final/Subsystem ==
  Display{,1..3,5..6} (6 alike) : Display
      settings: Format=bank
  Gain{1..3,5} (4 alike) : Gain
  Scope : Scope  NumInputPorts=4
  wires:
  [Wind_generation_power] -> Gain3/1
  [Active_Grid_Power] -> Scope/4, Display3/1
  [Reactive_Grid_Power] -> Display5/1
  [Reactive_Demand_Power] -> Gain5/1
  [Battery_power] -> Gain2/1
  [Active_Demand_Power] -> Gain1/1
  Gain3/1 -> Scope/1, Display/1
  Gain1/1 -> Display2/1, Scope/2
  Gain2/1 -> Display1/1, Scope/3
  Gain5/1 -> Display6/1

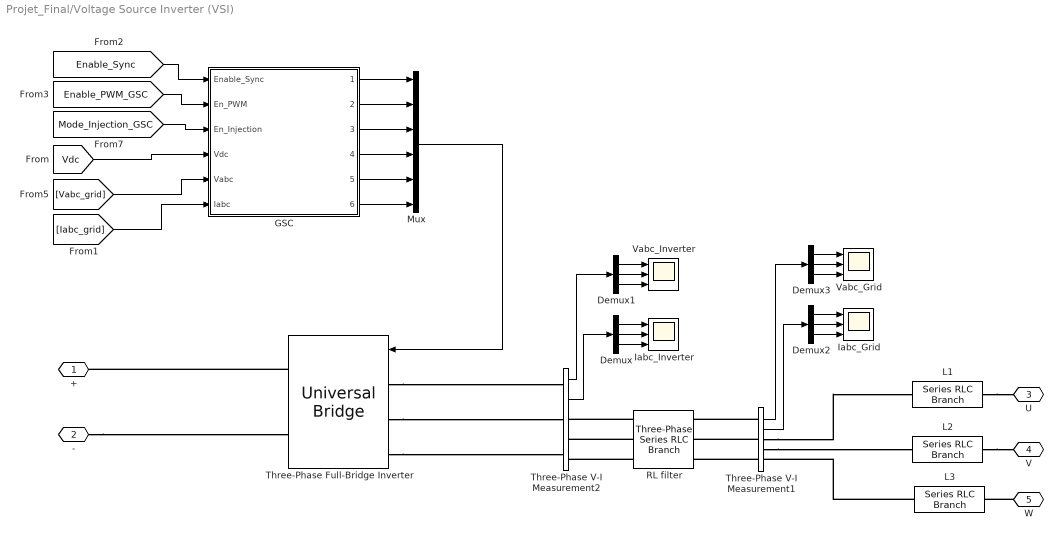
== system Projet_Final/Voltage Source Inverter (VSI) ==
  Demux{,1..3} (4 alike) : Demux  Outputs=3
  GSC : Subsystem
      settings: PortSchema="{\"entries\":[{\"content\":{\"sides\":[{\"content\":{},\"type\":\"ConnectorPlacement.EquallySpacedRectSide\",\"uuid\":\"68bdff09-e8ec-4d6d-b05e-55201ee357f5\"},{\"content\":{\"side\":\"RIGHT\"},\"type\":\"ConnectorPlacement.EquallySpacedRectSide\",\"uuid\":\"a14a2bca-9db8-408e-b5bf-8e3869a2fb13\"},{\"content\":{\"connectorIds\":[\"Out1\",\"Out2\",\"Out3\",\"Out4\",\"Out5\",\"Out6\"],\"side\":\"TOP\"},\"type\":\"ConnectorPlacement.EquallySpacedRectSide\",\"uuid\":\"600d12f1-b4e8-4864-955c-a539efb19c99\"},{\"content\":{\"connectorIds\":[\"In1\",\"In2\",\"In3\",\"In4\",\"In5\",\"In6\"],\"side\":\"BOTTOM\"},\"type\":\"ConnectorPlacement.EquallySpacedRectSide\",\"uuid\":\"cfcd8960-7e69-4555-b569-2db0e2e04180\"}]},\"type\":\"ConnectorPlacement.EquallySpacedConnector\",\"uuid\":\"05b2b3d9-6bdc-4d72-9457-a6c68afa543f\"}],\"packageUris\":[\"http://schema.mathworks.com/mf0/Connector/R2020b\"],\"version\":\"1.0\"}"
      mask Display: image('Cotroller.jpg', [0,0,0,0,70,70]);
  Iabc_Grid : Scope  NumInputPorts=3
  Iabc_Inverter : Scope  NumInputPorts=3
  L1 : spsSeriesRLCBranchLib/Series RLC Branch  LConnTagsString=__new0  RConnTagsString=__new0  BranchType=RL  Resistance=0.01  Inductance=1e-12  SetiL0=off  InitialCurrent=0  Capacitance=C_dc  Setx0=on  InitialVoltage=Vdc_ref  Measurements=None
  L2 : spsSeriesRLCBranchLib/Series RLC Branch  LConnTagsString=__new0  RConnTagsString=__new0  BranchType=RL  Resistance=0.01  Inductance=1e-12  SetiL0=off  InitialCurrent=0  Capacitance=C_dc  Setx0=on  InitialVoltage=Vdc_ref  Measurements=None
  L3 : spsSeriesRLCBranchLib/Series RLC Branch  LConnTagsString=__new0  RConnTagsString=__new0  BranchType=RL  Resistance=0.01  Inductance=1e-12  SetiL0=off  InitialCurrent=0  Capacitance=C_dc  Setx0=on  InitialVoltage=Vdc_ref  Measurements=None
  Mux : Mux  Inputs=6
  RL filter : spsThreePhaseSeriesRLCBranchLib/Three-Phase Series RLC Branch  LConnTagsString=A|B|C  RConnTagsString=A|B|C  BranchType=RL  Resistance=Rf  Inductance=Lf  Capacitance=1e-6  Measurements=None
  Three-Phase V-I Measurement1 : spsThreePhaseVIMeasurementLib/Three-Phase V-I Measurement  VoltageMeasurement=phase-to-ground  SetLabelV=off  LabelV=Vabc_Inverter  Vpu=off  VpuLL=off  CurrentMeasurement=yes  SetLabelI=off  LabelI=Iabc_Inverter  Ipu=off  Pbase=100e6  Vbase=500e3  OutputType=Complex  PhasorSimulation=off  PSBequivalent=0
  Three-Phase V-I Measurement2 : spsThreePhaseVIMeasurementLib/Three-Phase V-I Measurement  VoltageMeasurement=phase-to-ground  SetLabelV=off  LabelV=Vabc_Inverter  Vpu=off  VpuLL=off  CurrentMeasurement=yes  SetLabelI=off  LabelI=Iabc_Inverter  Ipu=off  Pbase=100e6  Vbase=500e3  OutputType=Complex  PhasorSimulation=off  PSBequivalent=0
  Three-Phase Full-Bridge Inverter : spsUniversalBridgeLib/Universal Bridge  Arms=3  SnubberResistance=1e7  SnubberCapacitance=inf  Device=IGBT / Diodes  Ron=1e-2  Lon=0  ForwardVoltages="[  0  0  ]"  ForwardVoltage=0  GTOparameters=[ 10e-6 , 20e-6 ]  IGBTparameters=[ 0 , 0 ]  Measurements=None  Measurements_2=None  converterType=Rectifier
  Vabc_Grid : Scope  NumInputPorts=3
  Vabc_Inverter : Scope  NumInputPorts=3
  + : PMIOPort  Side=Left
  - : PMIOPort  Port=2  Side=Left
  U : PMIOPort  Port=3  Side=Right
  V : PMIOPort  Port=4  Side=Right
  W : PMIOPort  Port=5  Side=Right
  wires:
  Three-Phase V-I Measurement2/2 -> Demux/1
  Demux/2 -> Iabc_Inverter/2
  Demux/1 -> Iabc_Inverter/1
  Demux/3 -> Iabc_Inverter/3
  Demux1/3 -> Vabc_Inverter/3
  Demux1/1 -> Vabc_Inverter/1
  Demux1/2 -> Vabc_Inverter/2
  Three-Phase V-I Measurement2/1 -> Demux1/1
  [Vdc] -> GSC/4(Vdc)
  Mux/1 -> Three-Phase Full-Bridge Inverter/1
  Three-Phase V-I Measurement1/1 -> Demux3/1
  Demux3/2 -> Vabc_Grid/2
  Demux3/1 -> Vabc_Grid/1
  Demux3/3 -> Vabc_Grid/3
  Demux2/3 -> Iabc_Grid/3
  Demux2/1 -> Iabc_Grid/1
  Demux2/2 -> Iabc_Grid/2
  Three-Phase V-I Measurement1/2 -> Demux2/1
  [Vabc_grid] -> GSC/5(Vabc)
  [Iabc_grid] -> GSC/6(Iabc)
  [Enable_PWM_GSC] -> GSC/2(En_PWM)
  [Mode_Injection_GSC] -> GSC/3(En_Injection)
  [Enable_Sync] -> GSC/1(Enable_Sync)
  GSC/1(" ") -> Mux/1
  GSC/2("  ") -> Mux/2
  GSC/3("   ") -> Mux/3
  GSC/4("    ") -> Mux/4
  GSC/5("     ") -> Mux/5
  GSC/6("      ") -> Mux/6
  connections:
  Three-Phase Full-Bridge Inverter/LConn3 -- Three-Phase V-I Measurement2/LConn3
  Three-Phase Full-Bridge Inverter/LConn2 -- Three-Phase V-I Measurement2/LConn2
  Three-Phase Full-Bridge Inverter/LConn1 -- Three-Phase V-I Measurement2/LConn1
  RL filter/LConn1 -- Three-Phase V-I Measurement2/RConn1
  RL filter/LConn2 -- Three-Phase V-I Measurement2/RConn2
  RL filter/LConn3 -- Three-Phase V-I Measurement2/RConn3
  Three-Phase V-I Measurement1/LConn1 -- RL filter/RConn1
  Three-Phase V-I Measurement1/LConn2 -- RL filter/RConn2
  Three-Phase V-I Measurement1/LConn3 -- RL filter/RConn3
  Three-Phase V-I Measurement1/RConn1 -- L1/LConn1
  Three-Phase V-I Measurement1/RConn2 -- L2/LConn1
  W/RConn1 -- L3/RConn1
  Three-Phase Full-Bridge Inverter/RConn1 -- +/RConn1
  -/RConn1 -- Three-Phase Full-Bridge Inverter/RConn2
  L2/RConn1 -- V/RConn1
  L1/RConn1 -- U/RConn1
  L3/LConn1 -- Three-Phase V-I Measurement1/RConn3

== system Projet_Final/Wind Generation 20 kw ==
  L1 : spsSeriesRLCBranchLib/Series RLC Branch  LConnTagsString=__new0  RConnTagsString=__new0  BranchType=RL  Resistance=0.01  Inductance=1e-6  SetiL0=off  InitialCurrent=0  Capacitance=C_dc  Setx0=on  InitialVoltage=Vdc_ref  Measurements=None
  L2 : spsSeriesRLCBranchLib/Series RLC Branch  LConnTagsString=__new0  RConnTagsString=__new0  BranchType=RL  Resistance=0.01  Inductance=1e-6  SetiL0=off  InitialCurrent=0  Capacitance=C_dc  Setx0=on  InitialVoltage=Vdc_ref  Measurements=None
  L3 : spsSeriesRLCBranchLib/Series RLC Branch  LConnTagsString=__new0  RConnTagsString=__new0  BranchType=RL  Resistance=0.01  Inductance=1e-6  SetiL0=off  InitialCurrent=0  Capacitance=C_dc  Setx0=on  InitialVoltage=Vdc_ref  Measurements=None
  PMSG : Subsystem
      settings: PortSchema="{\"entries\":[{\"content\":{\"sides\":[{\"content\":{\"connectorIds\":[\"Out1\",\"In1\"]},\"type\":\"ConnectorPlacement.EquallySpacedRectSide\",\"uuid\":\"3f25ae88-b85d-4aa8-83e0-c8881128a15f\"},{\"content\":{\"connectorIds\":[\"RConn1\",\"RConn2\",\"RConn3\"],\"side\":\"RIGHT\"},\"type\":\"ConnectorPlacement.EquallySpacedRectSide\",\"uuid\":\"21769176-b893-4bdb-b404-3c9a8a9ec7d7\"},{\"content\":{\"side\":\"TOP\"},\"type\":\"ConnectorPlacement.EquallySpacedRectSide\",\"uuid\":\"6b86daf7-1109-4b9d-a4e1-050e61d06be5\"}]},\"type\":\"ConnectorPlacement.EquallySpacedConnector\",\"uuid\":\"4237b530-1620-4b33-bc88-1364db079d0f\"}],\"packageUris\":[\"http://schema.mathworks.com/mf0/Connector/R2020b\"],\"version\":\"1.0\"}"
      mask Display: image('Machine.jpg');
  Wind Turbine : Subsystem
      settings: PortSchema="{\"entries\":[{\"content\":{\"sides\":[{\"content\":{},\"type\":\"ConnectorPlacement.EquallySpacedRectSide\",\"uuid\":\"46343f75-74e6-4f4c-9efc-4b43e6213925\"},{\"content\":{\"connectorIds\":[\"In1\",\"Out1\"],\"side\":\"RIGHT\"},\"type\":\"ConnectorPlacement.EquallySpacedRectSide\",\"uuid\":\"10880a8c-ba30-44f8-b93e-97455e8769b4\"},{\"content\":{\"side\":\"TOP\"},\"type\":\"ConnectorPlacement.EquallySpacedRectSide\",\"uuid\":\"fc9f6e01-6aae-438b-b3e4-23506a1fb9e3\"}]},\"type\":\"ConnectorPlacement.EquallySpacedConnector\",\"uuid\":\"29e446f6-be91-4db2-b818-9d2408c26281\"}],\"packageUris\":[\"http://schema.mathworks.com/mf0/Connector/R2020b\"],\"version\":\"1.0\"}"
      mask Display: image('Turbine.png');
  U1 : PMIOPort  Side=Right
  V1 : PMIOPort  Port=2  Side=Right
  W1 : PMIOPort  Port=3  Side=Right
  wires:
  PMSG/1(Omega_G) -> Wind Turbine/1(Omega)
  Wind Turbine/1(Tm) -> PMSG/1(Tm)
  connections:
  PMSG/RConn2 -- L2/LConn1
  W1/RConn1 -- L3/RConn1
  L1/LConn1 -- PMSG/RConn1
  L2/RConn1 -- V1/RConn1
  L3/LConn1 -- PMSG/RConn3
  U1/RConn1 -- L1/RConn1

== system Projet_Final/Active Rectifier/       ==
  note: Estimation de P_aéro Maximale
  note: Adaptive P&O
  Input2 : Inport
  Input : Inport  Port=2
  Input1 : Inport  Port=3
  Constant : Constant
  MATLAB Function2 : MATLAB Function  TreatAsAtomicUnit=on  SystemSampleTime=0.001
  MATLAB Function3 : MATLAB Function  TreatAsAtomicUnit=on  SystemSampleTime=0.001
  Mux : Mux  Inputs=2
  Mux1 : Mux  Inputs=2
  NOT1 : Logic  Operator=NOT  IconShape=distinctive  AllPortsSameDT=off  OutDataTypeStr=boolean
  Scope : Scope  NumInputPorts=5
  Omega_ref : Outport
  wires:
  Input2/1 -> MATLAB Function2/1(P_mes)
  MATLAB Function2/1(Omega_ref) -> Omega_ref/1
  Input/1 -> MATLAB Function3/1(V_vent)
  [Omega_G_ref] -> Mux/2
  [Omega_G] -> Mux/1
  Mux1/1 -> Scope/1
  Mux/1 -> Scope/2
  [Cp] -> Scope/3
  [Ta] -> Scope/4
  [wind_speed] -> Scope/5
  [Omega_ref_init] -> MATLAB Function2/3(Omega_Start)
  [Pa] -> Mux1/2
  Input1/1 -> NOT1/1
  MATLAB Function3/1(P_aero_ref) -> Mux1/1, MATLAB Function2/2(P_betz)
  NOT1/1 -> MATLAB Function2/4(Activation)

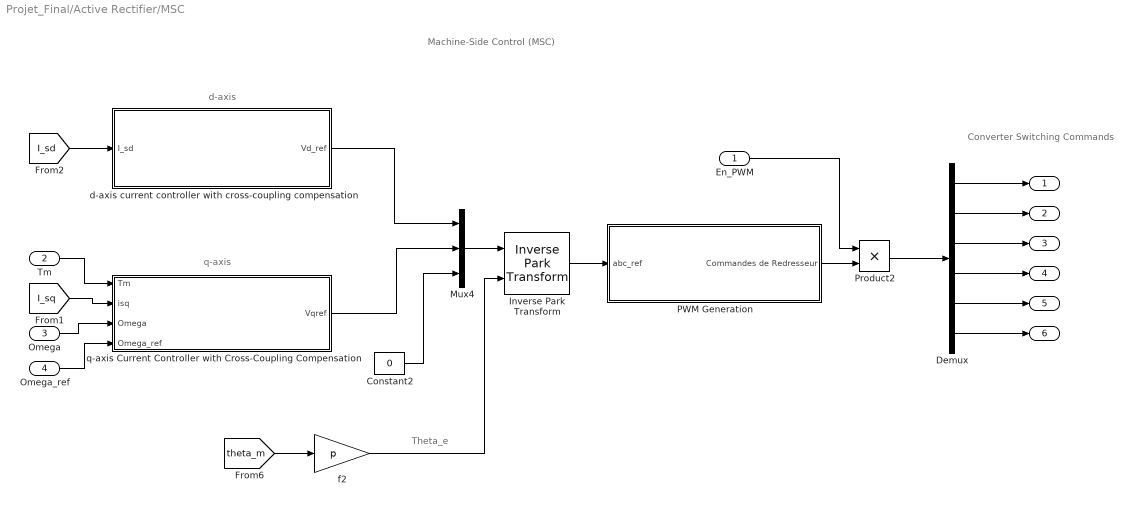
== system Projet_Final/Active Rectifier/MSC ==
  note: Converter Switching Commands
  note: q-axis
  note: d-axis
  note: Theta_e
  note: Machine-Side Control (MSC)
  En_PWM : Inport
  Tm : Inport  Port=2
  Omega : Inport  Port=3
  Omega_ref : Inport  Port=4
  Constant2 : Constant  Value=0
  Demux : Demux  Outputs=6
  Inverse Park Transform : eeTransforms/Inverse Park Transform  AxisAlignment=Q-axis  PowerInvariant=off
      settings: LibrarySourceBlock=|
      | ee_sl_lib/Mathematical
      | Transforms/Inverse
      | Park Transform
  Mux4 : Mux  Inputs=3
  PWM Generation : Subsystem
  Product2 : Product
  d-axis current controller with cross-coupling compensation : Subsystem
  f2 : Gain  Gain=p  SaturateOnIntegerOverflow=on  OutDataTypeStr=Inherit: Same as input  ParamDataTypeStr=Inherit: Same as input
  "q-axis Current Controller with Cross-Coupling Compensation " : Subsystem
  " " : Outport
  "  " : Outport  Port=2
  "   " : Outport  Port=3
  "    " : Outport  Port=4
  "     " : Outport  Port=5
  "       " : Outport  Port=6
  wires:
  Constant2/1 -> Mux4/3
  Inverse Park Transform/1 -> PWM Generation/1(abc_ref)
  [theta_m] -> f2/1
  d-axis current controller with cross-coupling compensation/1(Vd_ref) -> Mux4/1
  "q-axis Current Controller with Cross-Coupling Compensation "/1(Vqref) -> Mux4/2
  Product2/1 -> Demux/1
  f2/1 -> Inverse Park Transform/2
  Demux/1 -> " "/1
  Demux/2 -> "  "/1
  Demux/3 -> "   "/1
  Demux/4 -> "    "/1
  Demux/5 -> "     "/1
  Demux/6 -> "       "/1
  Mux4/1 -> Inverse Park Transform/1
  PWM Generation/1(Commandes de Redresseur) -> Product2/2
  Tm/1 -> "q-axis Current Controller with Cross-Coupling Compensation "/1(Tm)
  Omega/1 -> "q-axis Current Controller with Cross-Coupling Compensation "/3(Omega)
  Omega_ref/1 -> "q-axis Current Controller with Cross-Coupling Compensation "/4(Omega_ref)
  [I_sq] -> "q-axis Current Controller with Cross-Coupling Compensation "/2(isq)
  En_PWM/1 -> Product2/1
  [I_sd] -> d-axis current controller with cross-coupling compensation/1(I_sd)
